simulink model "P2_SIL_Model_Diag"  (R2016a)
settings: Solver=ode2  StartTime=0.0  StopTime=Cycle_End  RelTol=1e-3
undefined symbols (not defined in the file): air, APP1_OOR, APP2_OOR, APP_Conversion_IN, APP_Mismatch, bms_inletair_temp, bms_maxchargecurrent, bms_maxdischargecurrent, BMS_Notfallkuehlung, BPP_Flt, cal, clt, ClutchEngag, CrankRequest, dcdc, eng, Engine, EngOverTemp, ENGTRQ_MSMCH_Degraded_CP, ENGTRQ_MSMCH_ErrCritical_CP, ENGTRQ_MSMCH_LimpHome_CP, EngTrqMismatch, env, ess, ESS, ESSOverTemp, fd, FFD, g, gb, Grade, IMG, KeyPos_Flt, KeyPosition, lib_APP_Conversion_IN, lib_ESS_plant_V1_2, lib_OBC_Manager, LossCAN, max_vehicle_rad_air_flow, MCUOverTemp, mot, MotDirMismatch, MotOverTemp, MotTrqMismatch, mph2kph, mph2ms, NeutralGear, obc, OBC_Manager, ParkGear, PRNDL_Flt, ReverseGear, RFD, rho, ShiftLeverPosition, sigbuilder_block, Speed, t_amb, time, tloop ... (+2)
libraries: simulink x104, EC2_libraries x12, Diagnostic x11, lib_CANerror_Detect x3, Utility x1
(part 4 of 11)

== system P2_SIL_Model_Diag/Camaro Plant Model/On-Board Charger/Soft_OBC/NLG5_ERR ==
  Bus Creator : BusCreator  Inputs=34
  Constant{1..34} (34 alike) : Constant  Value=0
  NLG5_ERR : Outport
  wires:
  Constant34/1 -> Bus Creator/34  "NLG5_E_PL_MV"
  Constant33/1 -> Bus Creator/33  "NLG5_E_PL_BV"
  Constant32/1 -> Bus Creator/32  "NLG5_E_PL_IT"
  Constant31/1 -> Bus Creator/31  "NLG5_E_C_VOR"
  Constant30/1 -> Bus Creator/30  "NLG5_E_C_TX"
  Constant29/1 -> Bus Creator/29  "NLG5_E_C_RX"
  Constant28/1 -> Bus Creator/28  "NLG5_E_SDT_BT"
  Constant27/1 -> Bus Creator/27  "NLG5_E_SDT_BV"
  Constant26/1 -> Bus Creator/26  "NLG5_E_SDT_AH"
  Constant25/1 -> Bus Creator/25  "NLG5_E_SDT_CT"
  Constant24/1 -> Bus Creator/24  "NLG5_E_F_CRC"
  Constant23/1 -> Bus Creator/23  "NLG5_E_NV_CRC"
  Constant22/1 -> Bus Creator/22  "NLG5_E_ES_CRC"
  Constant21/1 -> Bus Creator/21  "NLG5_E_EP_CRC"
  Constant20/1 -> Bus Creator/20  "NLG5_E_WDT"
  Constant19/1 -> Bus Creator/19  "NLG5_E_INIT"
  Constant18/1 -> Bus Creator/18  "NLG5_E_C_TO"
  Constant17/1 -> Bus Creator/17  "NLG5_E_C_OFF"
  Constant16/1 -> Bus Creator/16  "NLG5_E_B_P"
  Constant15/1 -> Bus Creator/15  "NLG5_E_T_C"
  Constant14/1 -> Bus Creator/14  "NLG5_E_T_POW"
  Constant13/1 -> Bus Creator/13  "NLG5_E_T_DIO"
  Constant12/1 -> Bus Creator/12  "NLG5_E_T_TR"
  Constant11/1 -> Bus Creator/11  "NLG5_E_T_EXT1"
  Constant10/1 -> Bus Creator/10  "NLG5_E_T_EXT2"
  Constant9/1 -> Bus Creator/9  "NLG5_E_T_EXT3"
  Constant8/1 -> Bus Creator/8  "NLG5_E_OOV"
  Constant7/1 -> Bus Creator/7  "NLG5_E_MOV_I"
  Constant5/1 -> Bus Creator/6  "NLG5_E_MOV_II"
  Constant2/1 -> Bus Creator/3  "NLG5_E_P_MV"
  Constant3/1 -> Bus Creator/4  "NLG5_E_P_OM"
  Constant1/1 -> Bus Creator/2  "NLG5_E_OF"
  Constant6/1 -> Bus Creator/1  "NLG5_E_MF"
  Bus Creator/1 -> NLG5_ERR/1  "NLG5_ERR"
  Constant4/1 -> Bus Creator/5  "NLG5_E_SC"

== system P2_SIL_Model_Diag/Camaro Plant Model/On-Board Charger/Soft_OBC/NLG5_ST ==
  Bus Creator : BusCreator  Inputs=24
  Constant10 : Constant
  Constant11 : Constant
  Constant{3..5,7,15..24} (14 alike) : Constant  Value=0
  Constant9 : Constant
  EVSE_Voltage : Constant  Value=obc.plant.init.Level2ChargerVoltage
  EVSE_Voltage1 : Constant  Value=obc.plant.init.Level1ChargerVoltage
  Logical Operator : Logic  Operator=OR  AllPortsSameDT=off  OutDataTypeStr=boolean
  Relational Operator : RelationalOperator  Operator===  OutDataTypeStr=boolean
  Relational Operator1 : RelationalOperator  Operator===  OutDataTypeStr=boolean
  NLG5_ST : Outport
  wires:
  EVSE_Voltage1/1 -> Relational Operator1/2
  EVSE_Voltage/1 -> Relational Operator/2
  [NLG5_MV_ACT] -> Relational Operator1/1, Relational Operator/1
  Constant4/1 -> Bus Creator/5  "NLG5_S_FAN"
  Bus Creator/1 -> NLG5_ST/1  "NLG5_ST"
  Logical Operator/1 -> Bus Creator/1  "NLG5_S_CP_DT"
  Relational Operator/1 -> Bus Creator/2, Logical Operator/1  "NLG5_S_UM_II"
  Constant3/1 -> Bus Creator/4  "NLG5_S_EUM"
  Relational Operator1/1 -> Bus Creator/3, Logical Operator/2  "NLG5_S_UM_I"
  Constant5/1 -> Bus Creator/6  "NLG5_S_WAR"
  Constant7/1 -> Bus Creator/7  "NLG5_S_ERR"
  [NLG5_S_HE] -> Bus Creator/8  "NLG5_S_HE"
  Constant9/1 -> Bus Creator/9  "NLG5_S_L_PMAX"
  Constant10/1 -> Bus Creator/10  "NLG5_S_L_CP"
  Constant11/1 -> Bus Creator/11  "NLG5_S_L_PI"
  [NLG5_S_L_MC] -> Bus Creator/12  "NLG5_S_L_MC"
  [NLG5_S_L_OC] -> Bus Creator/13  "NLG5_S_L_OC"
  [NLG5_S_L_OV] -> Bus Creator/14  "NLG5_S_L_OV"
  Constant15/1 -> Bus Creator/15  "NLG5_S_BPD_II"
  Constant16/1 -> Bus Creator/16  "NLG5_S_BPD_I"
  Constant17/1 -> Bus Creator/17  "NLG5_S_L_T_BATT"
  Constant18/1 -> Bus Creator/18  "NLG5_S_L_T_TR"
  Constant19/1 -> Bus Creator/19  "NLG5_S_L_T_DIO"
  Constant20/1 -> Bus Creator/20  "NLG5_S_L_T_POW"
  Constant21/1 -> Bus Creator/21  "NLG5_S_L_T_CPRIM"
  Constant22/1 -> Bus Creator/22  "NLG5_S_L_MO_MAX"
  Constant23/1 -> Bus Creator/23  "NLG5_S_L_OC_MAX"
  Constant24/1 -> Bus Creator/24  "NLG5_S_L_MC_MAX"

== system P2_SIL_Model_Diag/Camaro Plant Model/On-Board Charger/Soft_OBC/NLG5_TEMP ==
  Bus Creator : BusCreator  Inputs=4
  NoiseAdd : Subsystem  AncestorBlock=EC2_libraries/NoiseAdd  mask{variance=0, seed=0}
  NoiseAdd1 : Subsystem  AncestorBlock=EC2_libraries/NoiseAdd  mask{variance=0, seed=0}
  NoiseAdd2 : Subsystem  AncestorBlock=EC2_libraries/NoiseAdd  mask{variance=0, seed=0}
  NLG5_TEMP : Outport
  wires:
  Bus Creator/1 -> NLG5_TEMP/1  "NLG5_TEMP"
  [NLG5_TEMP] -> Bus Creator/1  "NLG5_P_TMP"
  [NLG5_TEMP] -> NoiseAdd/1(In)  "NLG5_TMP_EXT1"
  [NLG5_TEMP] -> NoiseAdd2/1(In)  "NLG5_TMP_EXT3"
  [NLG5_TEMP] -> NoiseAdd1/1(In)  "NLG5_TEMP_EXT2"
  NoiseAdd/1(Out) -> Bus Creator/2  "NLG5_TMP_EXT1"
  NoiseAdd1/1(Out) -> Bus Creator/3  "NLG5_TMP_EXT2"
  NoiseAdd2/1(Out) -> Bus Creator/4  "NLG5_TMP_EXT3"

== system P2_SIL_Model_Diag/Camaro Plant Model/On-Board Charger/Soft_OBC/VoltageEnable ==
  OV_COM : Inport
  Logical Operator1 : Logic  AllPortsSameDT=off  OutDataTypeStr=boolean
  MaxOutVoltage : Constant  Value=obc.plant.init.Maximum_Voltage_Out
  MinMax1 : MinMax  Inputs=2
  MinOutVoltage : Constant  Value=obc.plant.init.Minimum_Voltage_Out
  Relational Operator : RelationalOperator  OutDataTypeStr=boolean
  Relational Operator1 : RelationalOperator  Operator=<=  OutDataTypeStr=boolean
  Relational Operator2 : RelationalOperator  Operator=>  OutDataTypeStr=boolean
  VoltageEnable : Outport
  tag scope: NLG5_S_L_OV=global
  wires:
  MinMax1/1 -> Relational Operator/1
  MaxOutVoltage/1 -> MinMax1/2, Relational Operator2/2
  OV_COM/1 -> MinMax1/1, Relational Operator2/1
  Relational Operator1/1 -> Logical Operator1/2
  Relational Operator/1 -> Logical Operator1/1
  MinOutVoltage/1 -> Relational Operator1/1
  Relational Operator2/1 -> [NLG5_S_L_OV]
  Logical Operator1/1 -> VoltageEnable/1
  [NLG5_OV_ACT] -> Relational Operator/2, Relational Operator1/2

== system P2_SIL_Model_Diag/Camaro Plant Model/Transmission1/Inputs/Analog_fromHCU ==
  Outputs : Outport
  wires:
  [Analog] -> Outputs/1

== system P2_SIL_Model_Diag/Camaro Plant Model/Transmission1/Inputs/CAN_fromHCU ==
  Outputs : Outport
  wires:
  [HCU_to_VEH_CAN] -> Outputs/1

== system P2_SIL_Model_Diag/Camaro Plant Model/Transmission1/Inputs/Digital_fromHCU ==
  Outputs : Outport
  wires:
  [Digital] -> Outputs/1

== system P2_SIL_Model_Diag/Camaro Plant Model/Transmission1/Soft TCM/6L45 Logic/Gearbox_Control.Shift_Schedule.PlotShiftSchedule ==
  f : TriggerPort  TriggerType=function-call  VariantControl=Variant
      settings: CopyFcn=Stateflow.SLINSF.SimulinkMan.removeBlockPreDeleteFcn  PreDeleteFcn=Stateflow.SLINSF.SimulinkMan.unsafePredeleteFcn
  Subsystem : Subsystem
      settings: OpenFcn=|
      | figure;
      | PlotGearShiftSchedule(Gearbox.L45.PedalPositions,Gearbox.L45.UpShiftSpeeds,Gearbox.L45.DownShiftSpeeds,'6L45')
      mask Display: disp('Plot')

== system P2_SIL_Model_Diag/Camaro Plant Model/Transmission1/Soft TCM/6L45 Logic/Gearbox_Control.Shift_Schedule.calc_down ==
  Gear : Inport
  APP : Inport  Port=2
  f : TriggerPort  TriggerType=function-call  VariantControl=Variant
      settings: CopyFcn=Stateflow.SLINSF.SimulinkMan.removeBlockPreDeleteFcn  PreDeleteFcn=Stateflow.SLINSF.SimulinkMan.unsafePredeleteFcn
  Calculate Downshift Threshold : Lookup2D  RowIndex=gb.ctrl.dmd.init.gear_dnshift.idx1_lin_accel  ColumnIndex=[2,3,4,5,6,7,8]  Table=gb.ctrl.dmd.init.gear_dnshift.map'  LookUpMeth=Interpolation-Use End Values
  down_th : Outport
  wires:
  APP/1 -> Calculate Downshift Threshold/1
  Gear/1 -> Calculate Downshift Threshold/2
  Calculate Downshift Threshold/1 -> down_th/1

== system P2_SIL_Model_Diag/Camaro Plant Model/Transmission1/Soft TCM/6L45 Logic/Gearbox_Control.Shift_Schedule.calc_up ==
  Gear : Inport
  APP : Inport  Port=2
  f : TriggerPort  TriggerType=function-call  VariantControl=Variant
      settings: CopyFcn=Stateflow.SLINSF.SimulinkMan.removeBlockPreDeleteFcn  PreDeleteFcn=Stateflow.SLINSF.SimulinkMan.unsafePredeleteFcn
  Calculate Upshift Threshold : Lookup2D  RowIndex=gb.ctrl.dmd.init.gear_upshift.idx1_lin_accel  ColumnIndex=[1,2,3,4,5,6,7]  Table=gb.ctrl.dmd.init.gear_upshift.map'  LookUpMeth=Interpolation-Use End Values
  up_th : Outport
  wires:
  Gear/1 -> Calculate Upshift Threshold/2
  APP/1 -> Calculate Upshift Threshold/1
  Calculate Upshift Threshold/1 -> up_th/1

== system P2_SIL_Model_Diag/Camaro Plant Model/Transmission1/Soft TCM/6L45 Logic/Torque_Converter_Control.calc_lockup ==
  Gear : Inport
  APP : Inport  Port=2
  f : TriggerPort  TriggerType=function-call  VariantControl=Variant
      settings: CopyFcn=Stateflow.SLINSF.SimulinkMan.removeBlockPreDeleteFcn  PreDeleteFcn=Stateflow.SLINSF.SimulinkMan.unsafePredeleteFcn
  Calculate Lockup Threshold : Lookup2D  RowIndex=cpl.ctrl.init.trqconv_lockup.idx1_lin_accel  ColumnIndex=cpl.ctrl.init.trqconv_lockup.idx2_gear  Table=cpl.ctrl.init.trqconv_lockup.map  LookUpMeth=Interpolation-Use End Values
  lockup_th : Outport
  wires:
  Gear/1 -> Calculate Lockup Threshold/2
  APP/1 -> Calculate Lockup Threshold/1
  Calculate Lockup Threshold/1 -> lockup_th/1

== system P2_SIL_Model_Diag/Camaro Plant Model/Transmission1/Soft TCM/6L45 Logic/Torque_Converter_Control.calc_unlock ==
  Gear : Inport
  APP : Inport  Port=2
  f : TriggerPort  TriggerType=function-call  VariantControl=Variant
      settings: CopyFcn=Stateflow.SLINSF.SimulinkMan.removeBlockPreDeleteFcn  PreDeleteFcn=Stateflow.SLINSF.SimulinkMan.unsafePredeleteFcn
  Calculate Unlock Threshold : Lookup2D  RowIndex=cpl.ctrl.init.trqconv_unlock.idx1_lin_accel  ColumnIndex=cpl.ctrl.init.trqconv_unlock.idx2_gear  Table=cpl.ctrl.init.trqconv_unlock.map  LookUpMeth=Interpolation-Use End Values
  unlock_th : Outport
  wires:
  Gear/1 -> Calculate Unlock Threshold/2
  APP/1 -> Calculate Unlock Threshold/1
  Calculate Unlock Threshold/1 -> unlock_th/1

== system P2_SIL_Model_Diag/Camaro Plant Model/Transmission1/Transmission Plant/ Actuators ==
  In1 : Inport
  Bus Selector : BusSelector  OutputSignals=TransEstGear,LockupCmd
  Out2 : Outport
  Out5 : Outport  Port=2
  wires:
  Bus Selector/2 -> Out5/1  "<LockupCmd>"
  Bus Selector/1 -> Out2/1  "<TransEstGear>"
  In1/1 -> Bus Selector/1

== system P2_SIL_Model_Diag/Camaro Plant Model/Transmission1/Transmission Plant/Gearbox ==
  TransEstGear : Inport
  gb_trq_in gb_inertia_in : Inport  Port=2
  gb_spd_out : Inport  Port=3
  Bus Creator : BusCreator  Inputs=2
  Bus Selector : BusSelector  OutputSignals=tc_trq_out,tc_inertia_out
  Gear : Lookup  InputValues=gb.plant.init.gear.idx1_shifter  Table=gb.plant.init.gear.idx2_gear  LookUpMeth=Interpolation-Use End Values  OutDataTypeStr=double  SaturateOnIntegerOverflow=on
  Inertia Calculation : Subsystem
  Memory : Memory
  Speed Calculation : Subsystem
  Torque calculation : Subsystem
  gear ratio table : Lookup  InputValues=gb.plant.init.ratio.idx1_gear  Table=gb.plant.init.ratio.map  LookUpMeth=Interpolation-Use End Values  SaturateOnIntegerOverflow=on
  gb_trq_out gb_inertia_out : Outport
  gb_spd_in : Outport  Port=2
  tag scope: gb_gear=global, gb_inertia_in=global, gb_inertia_out=global, gb_spd_in=global, gb_spd_out=global, gb_trq_in=global, gb_trq_out=global, gb_trq_ratio=global
  wires:
  TransEstGear/1 -> Memory/1
  Bus Selector/1 -> [gb_trq_in], Speed Calculation/3(torque input), Torque calculation/3(" input torque")  "<tc_trq_out>"
  Gear/1 -> Speed Calculation/1(gear number), [gb_gear], gear ratio table/1, Inertia Calculation/2(gear number), Torque calculation/2(gear number)
  Torque calculation/1(torque_out) -> Bus Creator/1, [gb_trq_out]  "gb_trq_out"
  gb_spd_out/1 -> Torque calculation/1(speed out), [gb_spd_out], Speed Calculation/2(spd out)
  gb_trq_in gb_inertia_in/1 -> Bus Selector/1
  Speed Calculation/1(Speed) -> [gb_spd_in], gb_spd_in/1
  Bus Selector/2 -> [gb_inertia_in], Inertia Calculation/1(Inertia_in), Speed Calculation/4(Inertia Input)  "<tc_inertia_out>"
  Inertia Calculation/1(Inertia) -> [gb_inertia_out], Bus Creator/2  "gb_inertia_out"
  Bus Creator/1 -> gb_trq_out gb_inertia_out/1
  gear ratio table/1 -> [gb_trq_ratio]
  Memory/1 -> Gear/1

== system P2_SIL_Model_Diag/Camaro Plant Model/Transmission1/Transmission Plant/Sensors ==
  In2 : Inport
  In3 : Inport  Port=2
  In4 : Inport  Port=3
  In5 : Inport  Port=4
  In6 : Inport  Port=5
  In7 : Inport  Port=6
  Bus Creator : BusCreator  Inputs=6
  Out1 : Outport
  wires:
  In7/1 -> Bus Creator/6  "TrnsOutShftTrq"
  In6/1 -> Bus Creator/5  "TrnsOutShftAngVel"
  In3/1 -> Bus Creator/2  "turbine_spd_rads"
  In5/1 -> Bus Creator/4  "tc_trq_out"
  In4/1 -> Bus Creator/3  "tc_trq_in"
  In2/1 -> Bus Creator/1  "impeller_spd_rads"
  Bus Creator/1 -> Out1/1

== system P2_SIL_Model_Diag/Camaro Plant Model/Transmission1/Transmission Plant/Torque Converter ==
  tc_lockup : Inport
  tc_shaft_in : Inport  Port=2
  tc_spd_out : Inport  Port=3
  Bus Creator : BusCreator  Inputs=2
  Bus Selector : BusSelector  OutputSignals=mot_trq_out,mot_inertia_out
  Inertia Calculation : Subsystem
  Speed Calculation : Subsystem
  Torque Calculation : Subsystem
  tc_shaft_out : Outport
  cpl_spd_in : Outport  Port=2
  tag scope: tc_spd_in=global, tc_spd_out=global, tc_trq_in=global, tc_trq_out=global
  wires:
  Torque Calculation/2(turbine_trq) -> Bus Creator/1, [tc_trq_out]  "tc_trq_out"
  Torque Calculation/1("impeller_trq ") -> Speed Calculation/4(impeller_trq)
  Speed Calculation/1(impeller spd) -> [tc_spd_in], Torque Calculation/1("impeller_spd "), cpl_spd_in/1
  Inertia Calculation/2(impeller inertia) -> Speed Calculation/2(impeller_inertia)
  Inertia Calculation/1(turbine inertia) -> Bus Creator/2  "tc_inertia_out"
  tc_spd_out/1 -> Torque Calculation/2(turbine_spd), Speed Calculation/1(turbine_spd), [tc_spd_out]
  tc_shaft_in/1 -> Bus Selector/1
  Bus Creator/1 -> tc_shaft_out/1
  Bus Selector/1 -> [tc_trq_in], Torque Calculation/4(input_trq)  "<mot_trq_out>"
  Bus Selector/2 -> Inertia Calculation/1(inertia in)  "<mot_inertia_out>"
  tc_lockup/1 -> Speed Calculation/3(lockup_cmd), Inertia Calculation/2(lockup cmd), Torque Calculation/3(lockup_cmd)  "tc_lockup_cmd"

== system P2_SIL_Model_Diag/Camaro Plant Model/Wheels/Force calculation/Blending ==
  note: State dependent blending
  input : Inport
  Control (state) : Inport  Port=2
  Fcn : Fcn  Expr=(u<xl)*yl + (xl<=u)*(u<xc)*((yc-yl)*(u-xl)/(xc-xl)+yl) + (xc<=u)*(u<xr)*((yc-yr)*(u-xr)/(xc-xr)+yr) + (xr<=u)*yr
  Product : Product  SaturateOnIntegerOverflow=on  InputSameDT=on  OutDataTypeStr=Inherit: Same as first input
  Out1 : Outport
  wires:
  input/1 -> Product/1
  Control (state)/1 -> Fcn/1
  Product/1 -> Out1/1
  Fcn/1 -> Product/2

== system P2_SIL_Model_Diag/Camaro Plant Model/Wheels/Force calculation/Rolling Resistance ==
  whl_spd : Inport
  grade : Inport  Port=2
  Add : Sum  Inputs=++++
  Add1 : Sum
  Divide : Product  Inputs=*/
  Product : Product  Inputs=3  SaturateOnIntegerOverflow=on  InputSameDT=on  OutDataTypeStr=Inherit: Same as first input
  Product{1..4,7} (5 alike) : Product  RndMeth=Zero
  Product5 : Product  Inputs=3  RndMeth=Zero
  Product6 : Product  Inputs=5  RndMeth=Zero
  Relational Operator : RelationalOperator  Operator=<=  InputSameDT=on
  Relational Operator1 : RelationalOperator  Operator=>  InputSameDT=on
  Sign : Signum
  Trigonometric Function : Trigonometry  Operator=cos
  env.init.gravity : Constant  Value=g
  radius : Gain  Gain=whl.plant.init.radius  SaturateOnIntegerOverflow=on  OutDataTypeStr=Inherit: Same as input  ParamDataTypeStr=Inherit: Same as input
  veh.plant.init.mass.total : Constant  Value=chas.plant.init.mass.body
  whl.plant.calc.weight_fraction_effective : Constant
  whl.plant.init.coeff_roll1 : Constant  Value=whl.plant.init.coeff_roll1
  whl.plant.init.coeff_roll2 : Constant  Value=whl.plant.init.coeff_roll2
  whl.plant.init.coeff_roll3 : Constant  Value=whl.plant.init.coeff_roll3
  whl.plant.init.coeff_roll4 : Constant  Value=whl.plant.init.coeff_roll4
  whl.plant.init.spd_thresh : Constant  Value=whl.plant.init.spd_thresh
  rolling resistence : Outport
  wires:
  Product/1 -> radius/1
  Sign/1 -> Product/3
  radius/1 -> rolling resistence/1  "tire rollig resistance"
  whl.plant.init.coeff_roll2/1 -> Product1/2
  whl.plant.init.coeff_roll3/1 -> Product2/2
  whl.plant.init.coeff_roll4/1 -> Product3/2
  whl_spd/1 -> Sign/1, Relational Operator/1, Product7/1, Relational Operator1/1, Product1/1, Product4/1, Product4/2, Product5/1, Product5/2, Product5/3
  Product4/1 -> Product2/1
  Product5/1 -> Product3/1
  Product3/1 -> Add/1
  Product2/1 -> Add/2
  Product1/1 -> Add/3
  whl.plant.init.coeff_roll1/1 -> Add/4
  Add/1 -> Product6/2
  veh.plant.init.mass.total/1 -> Product6/3
  env.init.gravity/1 -> Product6/4
  whl.plant.calc.weight_fraction_effective/1 -> Product6/5
  Trigonometric Function/1 -> Product6/1
  grade/1 -> Trigonometric Function/1
  Product6/1 -> Product/1
  whl.plant.init.spd_thresh/1 -> Relational Operator/2, Divide/2, Relational Operator1/2
  Relational Operator/1 -> Product7/2
  Product7/1 -> Divide/1
  Divide/1 -> Add1/1
  Relational Operator1/1 -> Add1/2
  Add1/1 -> Product/2

== system P2_SIL_Model_Diag/Controller/HSC/Camaro Fault Detection/Component Diagnostic ==
  note: Component Status Setting Rule
      | xxx_CompStatus could be 0, 1, 2 or 3
      | 0: component needs to be offline
      | 1: component needs torque plant to deliver creep torque
      | 2: component needs torque plant to limit maximum torque delivery
      | 3: component needs torque plant to operate normally
  note: Component Diagnostics
  Sensors1 : Inport
  Bus Creator : BusCreator  Inputs=9
  Clutch Component Diagnostic : Subsystem
  Driver Input Diagnostic : Subsystem
  ESS Component Diagnostic : Subsystem
  Engine Component Diagnostic : Subsystem
  Motor Component Diagnostic : Subsystem
  Override Clutch Status : Subsystem  AncestorBlock=Diagnostic/Camaro Diagnostic/Input Conversions/DriverInput_Conversions/Override APP (%)
  Override Driver Status : Subsystem  AncestorBlock=Diagnostic/Camaro Diagnostic/Input Conversions/DriverInput_Conversions/Override APP (%)
  Override ESS Status : Subsystem  AncestorBlock=Diagnostic/Camaro Diagnostic/Input Conversions/DriverInput_Conversions/Override APP (%)
  Override Engine Status : Subsystem  AncestorBlock=Diagnostic/Camaro Diagnostic/Input Conversions/DriverInput_Conversions/Override APP (%)
  Override MCU Status : Subsystem  AncestorBlock=Diagnostic/Camaro Diagnostic/Input Conversions/DriverInput_Conversions/Override APP (%)
  Override TCM Status : Subsystem  AncestorBlock=Diagnostic/Camaro Diagnostic/Input Conversions/DriverInput_Conversions/Override APP (%)
  Transmission Component Diagnostic : Subsystem
  Out2 : Outport
  wires:
  Sensors1/1 -> Driver Input Diagnostic/1(In1), ESS Component Diagnostic/1(In1), Bus Creator/9, Clutch Component Diagnostic/1(In1), Transmission Component Diagnostic/1(In1), Engine Component Diagnostic/1(In1), Motor Component Diagnostic/1(In1)  "RawSig"
  Bus Creator/1 -> Out2/1
  Driver Input Diagnostic/1(Out1) -> Override Driver Status/1(In1)  "Diver_CompDiag"
  ESS Component Diagnostic/1(Out1) -> Override ESS Status/1(In1)  "ESS_CompDiag"
  Engine Component Diagnostic/1(Out1) -> Override Engine Status/1(In1)  "ECM_CompDiag"
  Transmission Component Diagnostic/1(Out1) -> Override TCM Status/1(In1)  "TCM_CompDiag"
  Clutch Component Diagnostic/1(Out1) -> Override Clutch Status/1(In1)  "Clutch_Component"
  Override ESS Status/1(Out1) -> Bus Creator/2  "BMS_Status"
  Override Engine Status/1(Out1) -> Bus Creator/5  "ECM_Status"
  Override TCM Status/1(Out1) -> Bus Creator/7  "TCM_Status"
  Override Clutch Status/1(Out1) -> Bus Creator/8  "Clutch_Status"
  Override Driver Status/1(Out1) -> Bus Creator/1  "Driver_Input_Status"
  Engine Component Diagnostic/2(Out2) -> Bus Creator/6
  Motor Component Diagnostic/1(Out1) -> Override MCU Status/1(In1)  "MCU_CompDiag"
  Override MCU Status/1(Out1) -> Bus Creator/3  "MCU_Status"
  Motor Component Diagnostic/2(Out2) -> Bus Creator/4

== system P2_SIL_Model_Diag/Controller/HSC/Camaro Fault Detection/Input Conversions ==
  note: Input Conversions and Override Switches
  note: These subsystems convert variable types to match those used in the
      | supervisor. In addition, override switches installed on each signal can
      | be used to manually override and signal for testing purposes
  RawSig : Inport
  BMS_Conversions : Subsystem
  Bus Creator : BusCreator  Inputs=7
  Clutch_Conversions : Subsystem
  DriverInput_Conversions : Subsystem
  ECM_Conversions : Subsystem
  MCU_Conversions : Subsystem
  TCM_Conversions : Subsystem
  VehSig : Outport
  wires:
  DriverInput_Conversions/1(Out1) -> Bus Creator/1
  Bus Creator/1 -> VehSig/1  "InputConvAndOvrd"
  MCU_Conversions/1(Out1) -> Bus Creator/3
  BMS_Conversions/1(Out1) -> Bus Creator/2
  RawSig/1 -> DriverInput_Conversions/1(In1), BMS_Conversions/1(In1), Clutch_Conversions/1(In1), Bus Creator/7, TCM_Conversions/1(In1), ECM_Conversions/1(In1), MCU_Conversions/1(In1)  "RawSig"
  ECM_Conversions/1(Out1) -> Bus Creator/4
  TCM_Conversions/1(Out1) -> Bus Creator/5
  Clutch_Conversions/1(Out1) -> Bus Creator/6

== system P2_SIL_Model_Diag/Controller/HSC/Camaro Fault Detection/Signal Diagnostic ==
  note: Signal Valid Setting Rule
      | xxx_yyy_[z]_SigValid could be 0 or 1
      | 0: signal invalid
      | 1: signal vaild
  note: Signal Naming Rule
      | Example: xxx_yyy_[z]_SigValid
      | xxx: source of the signal (Drv, Clu, BCM, ECM, TCM, BMS and MCU)
      | yyy: description of the signal
      | z: unit of the signal (V, A, Nm, m/s, %, 01, 0123, etc.)
  note: These subsystems evaluate each signal for proper value range and other checks
  note: Signal Diagnostics
  VehSig : Inport
  Bus Creator : BusCreator  Inputs=6
  Clutch Signal Diagnostic : Subsystem  AncestorBlock=Diagnostic/Camaro Diagnostic/Signal Diagnostic/Transmission Signal Diagnostic
  Driver Signal Diagnostic : Subsystem
  ESS Signal Diagnostic : Subsystem
  Engine Signal Diagnostic : Subsystem
  Motor Signal Diagnostic : Subsystem
  Transmission Signal Diagnostic : Subsystem
  Out2 : Outport
  wires:
  VehSig/1 -> Driver Signal Diagnostic/1(Sensors1), ESS Signal Diagnostic/1(Sensors1), Motor Signal Diagnostic/1(Sensors1), Clutch Signal Diagnostic/1(Sensors1), Transmission Signal Diagnostic/1(Sensors1), Engine Signal Diagnostic/1(Sensors1)
  Driver Signal Diagnostic/1(Driver_SigDiag) -> Bus Creator/1  "Driver_SigDiag"
  ESS Signal Diagnostic/1(ESS_SigDiag) -> Bus Creator/2  "ESS_SigDiag"
  Motor Signal Diagnostic/1(Motor_SigDiag) -> Bus Creator/3  "Motor_SigDiag"
  Engine Signal Diagnostic/1(Engine_SigDiag) -> Bus Creator/4  "Engine_SigDiag"
  Transmission Signal Diagnostic/1(Out2) -> Bus Creator/5  "Transmission_SigDiag"
  Bus Creator/1 -> Out2/1  "SignalDiag"
  Clutch Signal Diagnostic/1(Out2) -> Bus Creator/6  "Clutch_SigDiag"

== system P2_SIL_Model_Diag/Controller/HSC/Camaro Fault Detection/Signal Generator  ==
  note: Signal Generator
  BCM_APM_OBC_CANFault : lib_CANerror_Detect/CAN_Error_Detection/BCM_APM_OBC_CANFault  Commented=on
  BMS_Signals : Subsystem
  Bus Creator2 : BusCreator  Inputs=6
  Clutch_Signals : Subsystem
  Driver_Signals : Subsystem
  EBCM_BodyCM_CANFault : lib_CANerror_Detect/CAN_Error_Detection/EBCM_BodyCM_CANFault  Commented=on
  ECM_Signals : Subsystem
  ECM_TCM_CANFault : lib_CANerror_Detect/CAN_Error_Detection/ECM_TCM_CANFault  Commented=on
  MCU_Signals : Subsystem
  TCM_Signals : Subsystem
  Out1 : Outport
  wires:
  [BMS_Signals] -> Bus Creator2/1
  [Driver_Signals] -> Bus Creator2/2
  Bus Creator2/1 -> Out1/1
  [MCU_Signals] -> Bus Creator2/3
  [ECM_Signals] -> Bus Creator2/4
  [TCM_Signals] -> Bus Creator2/5
  [Clutch_Signals] -> Bus Creator2/6
  EBCM_BodyCM_CANFault/1 -> ?
  ECM_TCM_CANFault/1 -> ?
  BCM_APM_OBC_CANFault/1 -> ?

== system P2_SIL_Model_Diag/Controller/HSC/Camaro Fault Detection/SystemDiag ==
  note: 0: SystemStatus: Offline
      | 1: SystemStatus Online
      | 2: SystemStatus Limited
  note: Powertrain Diagnostics
  note: These subsystems evaluate each powertrain to determine
      | the level of functionality allowed based on each of its components.
  In1 : Inport
  Bus Creator : BusCreator  Inputs=4
  Combined_SystemDiagnostics : Subsystem  Commented=through
  eSystemDiagnostics : Subsystem
  iceSystemDiagnostics : Subsystem
  Out1 : Outport
  wires:
  eSystemDiagnostics/1(Out1) -> Bus Creator/1
  Bus Creator/1 -> Out1/1  "SystemDiag"
  In1/1 -> eSystemDiagnostics/1(In1), iceSystemDiagnostics/1(In1), Bus Creator/4  "CompSig"
  iceSystemDiagnostics/1(Out1) -> Bus Creator/2

== system P2_SIL_Model_Diag/Controller/HSC/Driver_Requests/APP_BPP to DrvIntndAxlTrq1 ==
  note: //*cal.RWD.CreepTrqEnableBPP*//
  note: $Author: fj4499 $
      | $Rev: 577 $
      | $Date: 2016-09-19 08:53:15 -0500 (Mon,19 Sep 2016) $
  Sensors : Inport
  Abs : Abs
  Bus Creator : BusCreator  Inputs=3
  Bus Selector : BusSelector  OutputSignals=from_Analog.drv_APP_req_[%],from_CAN.fromVEH_CAN.from_TCM.Ratio,from_CAN.fromVEH_CAN.from_BCM.BrkPdlPos,from_CAN.fromEBCAN.from_ECM.VehSpdAvgDrvn,from_CAN.fromHV_CAN.from_MCU.D2_Motor_Speed
  Compare To Constant1 : simulink/Logic and Bit Operations/Compare To Constant  relop=>=  const=10  OutDataTypeStr=boolean
  Constant : Constant  Value=0
  Constant2 : Constant  Value=0
  MotorCreepTrq : Lookup  InputValues=cal.RWD.CreepTrq.idx1_spd  Table=cal.RWD.CreepTrq.idx2_trq
  Post Driver Intnded Axle Torque : Subsystem
  Scope : Scope
  Sum : Sum
  Sum1 : Sum
  Switch1 : Switch  Threshold=cal.Regen.MinMotSpd
  Switch2 : Switch  Criteria=u2 > Threshold  Threshold=1
  Switch3 : Switch  Threshold=1
  IntndAxlTrq : Outport
  IntndAxlTrqStatus : Outport  Port=2
  wires:
  Constant/1 -> Sum/1, Bus Creator/2  "BrkIntndAxlTrq"
  Abs/1 -> Switch1/2
  Bus Creator/1 -> IntndAxlTrqStatus/1
  Switch1/1 -> IntndAxlTrq/1
  Bus Selector/3 -> Compare To Constant1/1  "<BrkPdlPos>"
  Sum/1 -> Switch1/1, Bus Creator/1  "FullDrvIntndAxlTrq"
  Sensors/1 -> Bus Selector/1
  Post Driver Intnded Axle Torque/1(DrvIntndAxlTrq) -> Switch2/1, Sum1/1  "PostDrvIntndAxlTrq"
  Bus Selector/1 -> Post Driver Intnded Axle Torque/1(APP)  "<drv_APP_req_[%]>"
  Bus Selector/5 -> Abs/1  "<D2_Motor_Speed>"
  MotorCreepTrq/1 -> Switch3/3
  Sum1/1 -> Switch2/3
  Switch2/1 -> Scope/1, Switch1/3, Bus Creator/3, Sum/2  "DrvIntndAxlTrq"
  Bus Selector/4 -> MotorCreepTrq/1  "<VehSpdAvgDrvn>"
  Switch3/1 -> Sum1/2  "MotAxlCrpTrq"
  Compare To Constant1/1 -> Switch3/2
  Constant2/1 -> Switch3/1
  Bus Selector/2 -> Post Driver Intnded Axle Torque/2(TransGearRatio)  "<Ratio>"
  [mode] -> Post Driver Intnded Axle Torque/3(Mode), Switch2/2

== system P2_SIL_Model_Diag/Controller/HSC/Driver_Requests/APP_BPP to DrvIntndAxlTrq2 ==
  note: $Author: fj4499 $
      | $Rev: 577 $
      | $Date: 2016-09-19 08:53:15 -0500 (Mon,19 Sep 2016) $
  Sensors : Inport
  Bus Selector : BusSelector  OutputSignals=from_Analog.drv_APP_req_[%]
  Bus Selector1 : BusSelector  OutputSignals=DrvIntndAxlTrq
  Post Driver Intnded Axle Torque : Subsystem
  IntndAxlTrq : Outport
  wires:
  Bus Selector/1 -> Post Driver Intnded Axle Torque/1(APP)  "<drv_APP_req_[%]>"
  Sensors/1 -> Bus Selector/1
  [mode] -> Post Driver Intnded Axle Torque/3(Mode)
  Post Driver Intnded Axle Torque/1(DrvIntndAxlTrq) -> Bus Selector1/1
  Bus Selector1/1 -> IntndAxlTrq/1  "<DrvIntndAxlTrq>"
  [gb_trq_ratio] -> Post Driver Intnded Axle Torque/2(TransGearRatio)

== system P2_SIL_Model_Diag/Controller/HSC/Driver_Requests/Vehicle_Shutdown ==
  note: $Author: eo1000 $
      | $Rev: 509 $
      | $Date: 2014-01-13 11:43:00 -0500 (Mon, 13 Jan 2014) $
  note: Make sure PD is sent before components are disabled
  note: Key Position
      | KeyOFF: 0
      | KeyAccessory: 1
      | KeyIgnition: 2
      | KeyCrank = 3
  note: HCU Init: HCUStatus = 0;
      | Waiting Key OFF Cmd: HCUStatus = 1;
      | USB Diag Performed: HCUStatus = 2;
      | ECUs are off: HCUStatus = 3
      | CAN Off Cmd: HCUStatus = 4;
      | HCU Off Cmd: HCUStatus = 5;
  Sensors : Inport
  Diagnostics : Inport  Port=2
  Bus Selector : BusSelector  OutputSignals=from_CAN.fromVEH_CAN.from_BCM.SysPwrMd,from_Analog.EVSEPlugged
  Components Disabled : Subsystem
  Constant : Constant  Value=cal.Time.DiagUSB
  Gain2 : Gain  Gain=1/tloop
  HCU_Shutdown : Stateflow chart  TreatAsAtomicUnit=on
  HCUONCmd : Outport
  HCUStatus : Outport  Port=2
  Components_Disabled : Outport  Port=3
  wires:
  Bus Selector/2 -> HCU_Shutdown/4(Plugged)  "<EVSEPlugged>"
  HCU_Shutdown/1(HCUStatus) -> HCUStatus/1
  Sensors/1 -> Bus Selector/1, Components Disabled/1(Sensors)
  Components Disabled/1(Comp_Disabled) -> Components_Disabled/1, HCU_Shutdown/1(DisableComponents)
  Constant/1 -> Gain2/1
  Bus Selector/1 -> HCU_Shutdown/3(Key_Position)  "<SysPwrMd>"
  HCU_Shutdown/2(HCU_ON) -> HCUONCmd/1  "HCUONCmd"
  Gain2/1 -> HCU_Shutdown/2(DiagUSBTimerMax)
  Diagnostics/1 -> Components Disabled/2(Diagnostics)

== system P2_SIL_Model_Diag/Controller/HSC/Driver_Requests/Vehicle_Startup ==
  note: $Author: eo1000 $
      | $Rev: 294 $
      | $Date: 2013-11-14 10:23:49 -0500 (Thu, 14 Nov 2013) $
  note: DriverDoor <DOAjrSwAtv>
      | Open: 1
      | Close: 0
  note: SysPwrMd (EC3)
      | 0 - Off
      | 1 -  Accessory
      | 2 - Run
      | 3 - Crank Request
  Sensors : Inport
  Bus Creator : BusCreator  Inputs=2
  Enable Propulsion : Subsystem  RequirementInfo={'other' 'HCU_Requirements.xlsx' '@Simulink_requirement_item_9' 'true' 'Check if the conditions are true to allow regular or emergency (when in highway traffic) propulsion system activation ' '' } %GIDa_dfd30209_921a_4d0b_a7c1_96ecad5085d2
  Vehicle_Startup_Signals : Outport
  wires:
  Bus Creator/1 -> Vehicle_Startup_Signals/1
  Sensors/1 -> Enable Propulsion/1(Sensors)
  Enable Propulsion/1(StartVehEnable) -> Bus Creator/1  "EnablePrplsn"
  Enable Propulsion/2(EnablePrplsnStatus) -> Bus Creator/2  "EnablePrplsnStatus"

== system P2_SIL_Model_Diag/Controller/HSC/Powertrain Manager/HV Manager ==
  note: //OBC status to be coming from Diagnostic later//
  note: //add OBC charge limits//
  Sensors : Inport
  Controls : Inport  Port=2
  APM_Manager : Subsystem  Commented=on
  BMS_Manager : Subsystem
  OBC_Manager : Subsystem  AncestorBlock=lib_OBC_Manager/OBC_Manager
  BMS_CAN : Outport
  HV_BUS_Status : Outport  Port=2
  OBC_CAN : Outport  Port=3
  OBC_Status : Outport  Port=4
  BMS_Digital : Outport  Port=5
  APM_CAN : Outport  Port=6
  APM_Status : Outport  Port=7
  wires:
  BMS_Manager/2(HV_BUS_Status) -> [HV_BUS_Status], HV_BUS_Status/1  "HV_BUS_Status"
  Sensors/1 -> BMS_Manager/1(Sensors), OBC_Manager/2(Sensors)
  [HV_BUS_Status] -> OBC_Manager/1(HV_Status)
  OBC_Manager/1(OBC CAN) -> OBC_CAN/1
  OBC_Manager/2(OBC Status) -> OBC_Status/1
  Controls/1 -> BMS_Manager/2(Controls)
  BMS_Manager/1(BMS CAN) -> BMS_CAN/1
  BMS_Manager/3(BMS Digital) -> BMS_Digital/1
  [HV_BUS_Status] -> APM_Manager/1(HV_Status)
  APM_Manager/1(APM Controls) -> APM_CAN/1
  APM_Manager/2(APM Status) -> APM_Status/1

== system P2_SIL_Model_Diag/Controller/HSC/Powertrain Manager/Output Conversion ==
  In1 : Inport
  In2 : Inport  Port=2
  In3 : Inport  Port=3
  In4 : Inport  Port=4
  In5 : Inport  Port=5
  In6 : Inport  Port=6
  Bus Creator : BusCreator  Inputs=14
  Bus Creator1 : BusCreator  Inputs=7
  Bus Selector2 : BusSelector  OutputSignals=powerMode,closeMaincReq,EnablePrplsn,ClutchEngage,EngAppReq,EngOnReq,MtrTrqCmd,EnableInverter,EngTrqCmd,HV_req,SysPwrMd_0_3,TrnsShftLvrPos,VehSpdAvgDrvn_kph,AccPos_Perc
  Data Type Conversion{,1..3,5..13} (13 alike) : DataTypeConversion
  Memory : Memory
  Memory1 : Memory
  Memory2 : Memory
  Out1 : Outport
  wires:
  In1/1 -> [BMS_CAN]
  In2/1 -> [OBC_CAN]
  In4/1 -> Bus Selector2/1
  Bus Selector2/1 -> Memory/1  "<powerMode>"
  Bus Selector2/2 -> Memory1/1  "<closeMaincReq>"
  Bus Selector2/3 -> Data Type Conversion2/1  "<EnablePrplsn>"
  Bus Selector2/4 -> Data Type Conversion3/1  "<ClutchEngage>"
  Bus Selector2/6 -> Data Type Conversion5/1  "<EngOnReq>"
  Bus Selector2/7 -> Data Type Conversion6/1  "<MtrTrqCmd>"
  Bus Selector2/8 -> Data Type Conversion7/1  "<EnableInverter>"
  Bus Selector2/9 -> Data Type Conversion8/1  "<EngTrqCmd>"
  Bus Selector2/10 -> Data Type Conversion9/1  "<HV_req>"
  Bus Selector2/11 -> Memory2/1  "<SysPwrMd_0_3>"
  Data Type Conversion1/1 -> Bus Creator/2  "MO_BMS_Sollmodus"
  Data Type Conversion2/1 -> Bus Creator/3  "EnablePrplsn"
  Data Type Conversion3/1 -> Bus Creator/4  "ClutchEngage"
  Bus Selector2/5 -> Bus Creator/5  "<EngAppReq>"
  Data Type Conversion6/1 -> Bus Creator/7  "Torque_Command"
  Data Type Conversion7/1 -> Bus Creator/8  "Inverter_Enable"
  Data Type Conversion8/1 -> Bus Creator/9  "EngTrqCmd"
  Data Type Conversion9/1 -> Bus Creator/10  "HV_req"
  Data Type Conversion10/1 -> Bus Creator/11  "SysPwrMd"
  Data Type Conversion/1 -> Bus Creator/1  "powerMode"
  In3/1 -> [MCU_CAN]
  Data Type Conversion5/1 -> Bus Creator/6  "EngOnReq"
  Bus Creator1/1 -> Out1/1
  [BMS_CAN] -> Bus Creator1/1
  [OBC_CAN] -> Bus Creator1/2
  [MCU_CAN] -> Bus Creator1/3
  Bus Creator/1 -> Bus Creator1/4  "Controls"
  In5/1 -> Bus Creator1/5
  Bus Selector2/12 -> Data Type Conversion11/1  "<TrnsShftLvrPos>"
  Data Type Conversion11/1 -> Bus Creator/12  "ShftLvrPos"
  Bus Selector2/13 -> Data Type Conversion12/1  "<VehSpdAvgDrvn_kph>"
  Data Type Conversion12/1 -> Bus Creator/13  "VehSpdAvgDrvn_kph"
  Bus Selector2/14 -> Data Type Conversion13/1  "<AccPos_Perc>"
  Data Type Conversion13/1 -> Bus Creator/14  "AccPos_Perc"
  In6/1 -> Bus Creator1/6
  Memory/1 -> Data Type Conversion/1
  Memory1/1 -> Data Type Conversion1/1
  Memory2/1 -> Data Type Conversion10/1
  [ecm_CAN] -> Bus Creator1/7

== system P2_SIL_Model_Diag/Controller/HSC/Powertrain Manager/PowertrainSUSD ==
  note: //RWD.MaxShtdwnCurrent//
  note: //cal.Time.MCU.Restart.Time//
  note: //cal.Time.MCU.InvrtrRspns//
  HV_Bus_Status : Inport
  Sensors : Inport  Port=2
  Control : Inport  Port=3
  Bus Creator : BusCreator  Inputs=2
  Bus Creator1 : BusCreator  Inputs=4
  Bus Creator2 : BusCreator  Inputs=3
  Bus Selector : BusSelector  OutputSignals=from_CAN.fromHV_CAN.from_MCU.D6_Inverter_Enable_State,from_CAN.fromHV_CAN.from_MCU.D4_DC_Bus_Current
  Bus Selector1 : BusSelector  OutputSignals=ReadyToDrive,ReadyToCharge,HV Discharge
  Bus Selector2 : BusSelector  OutputSignals=EnableInverter
  Constant1 : Constant
  Constant2 : Constant  Value=0.5
  Constant3 : Constant
  Constant6 : Constant
  Crank Engine : Subsystem
  Data Type Conversion : DataTypeConversion  OutDataTypeStr=boolean
  Data Type Conversion1 : DataTypeConversion  OutDataTypeStr=boolean
  Data Type Conversion2 : DataTypeConversion  OutDataTypeStr=double
  From1 : From  Commented=on  GotoTag=Driver_Request  TagVisibility=global
  Motor Wake up / Shutdown : Stateflow chart  AncestorBlock=lib_PowertrainWUSD_Manager/PowertrainSUSD_Manager/Motor Wake up // Shutdown  TreatAsAtomicUnit=on
  Terminator : Terminator
  Terminator1 : Terminator
  Terminator2 : Terminator
  MCU_CAN : Outport
  MCU_Status : Outport  Port=2
  tag scope: ecm_CAN=global
  wires:
  Constant2/1 -> Motor Wake up / Shutdown/6(MaxShtdwnCrnt)
  Constant1/1 -> Motor Wake up / Shutdown/4(Inverter_Response_Time)
  Constant6/1 -> Motor Wake up / Shutdown/5(Restart_Time)
  Bus Selector/2 -> Motor Wake up / Shutdown/8(Motor_Current)  "<D4_DC_Bus_Current>"
  Motor Wake up / Shutdown/5(Inverter_Discharge) -> Data Type Conversion2/1
  Sensors/1 -> Crank Engine/1(Sensors), Bus Selector/1
  Bus Selector/1 -> Data Type Conversion1/1  "<D6_Inverter_Enable_State>"
  Data Type Conversion1/1 -> Motor Wake up / Shutdown/7(Inverter_Enabled)
  Bus Selector1/1 -> Motor Wake up / Shutdown/1(RdyToDrv)  "<ReadyToDrive>"
  Bus Selector1/2 -> Motor Wake up / Shutdown/2(RdyToChg)  "<ReadyToCharge>"
  Bus Selector1/3 -> Motor Wake up / Shutdown/3(HVDischarge)  "<HV Discharge>"
  Bus Creator/1 -> MCU_CAN/1  "MCU_CAN"
  HV_Bus_Status/1 -> Bus Selector1/1
  Data Type Conversion/1 -> Motor Wake up / Shutdown/9(CAN_Acc)
  Constant3/1 -> Data Type Conversion/1
  Motor Wake up / Shutdown/1(MCU_State) -> Bus Creator1/1  "MCU_State"
  Motor Wake up / Shutdown/2(MCU_ShtdwnRdy) -> Bus Creator1/2  "MCU_ShtdwnRdy"
  Motor Wake up / Shutdown/3(MCUFault) -> Bus Creator1/3  "MCUFault"
  Bus Creator1/1 -> MCU_Status/1  "MCU_Status"
  Control/1 -> Bus Selector2/1, Crank Engine/2(Control)
  Crank Engine/1(EngStatus) -> Bus Creator2/1, Terminator/1
  Crank Engine/2(EngCrankCmd) -> Bus Creator2/2, Terminator1/1
  Crank Engine/3(SysPwrMdOut) -> Bus Creator2/3, Terminator2/1
  Data Type Conversion2/1 -> Bus Creator/1  "Inverter_Discharge"
  Motor Wake up / Shutdown/6(Inverter_Enable) -> Bus Creator/2  "Inverter_Enable"
  Motor Wake up / Shutdown/4(MCU_Wake) -> Bus Creator1/4  "MCU Wake"
  Bus Selector2/1 -> Motor Wake up / Shutdown/10(EnableInverter)  "<EnableInverter>"
  Bus Creator2/1 -> [ecm_CAN]

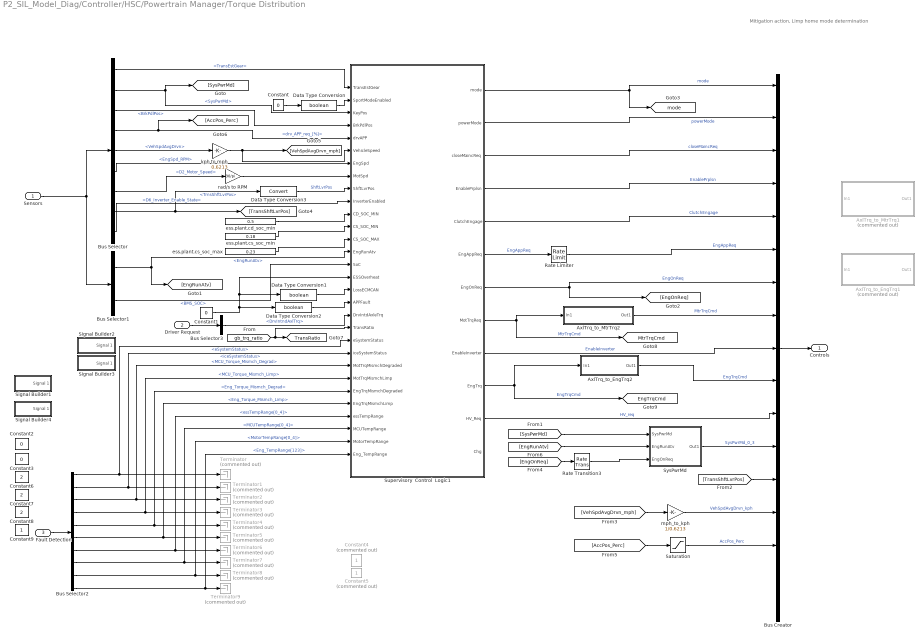
== system P2_SIL_Model_Diag/Controller/HSC/Powertrain Manager/Torque Distribution ==
  note: Mitigation action, Limp home mode determination
  Sensors : Inport
  Driver Request : Inport  Port=2
  Fault Detection : Inport  Port=3
  AxlTrq_to_EngTrq1 : Subsystem  Commented=on
  AxlTrq_to_EngTrq2 : Subsystem
  AxlTrq_to_MtrTrq1 : Subsystem  Commented=on
  AxlTrq_to_MtrTrq2 : Subsystem
  Bus Creator : BusCreator  Inputs=17
  Bus Selector : BusSelector  OutputSignals=from_CAN.fromVEH_CAN.from_TCM.TransEstGear,from_CAN.fromVEH_CAN.from_BCM.SysPwrMd,from_CAN.fromVEH_CAN.from_BCM.BrkPdlPos,from_Analog.drv_APP_req_[%],from_CAN.fromEBCAN.from_ECM.VehSpdAvgDrvn,from_CAN.fromEBCAN.from_ECM.EngSpd_RPM,from_CAN.fromHV_CAN.from_MCU.D2_Motor_Speed,from_CAN.fromVEH_CAN.from_TCM.TrnsShftLvrPos,from_CAN.fromHV_CAN.from_MCU.D6_Inverter_Enable_State
  Bus Selector1 : BusSelector  OutputSignals=from_CAN.fromEBCAN.from_ECM.EngRunAtv,from_CAN.fromHV_CAN.from_BMSHybrid.BMS_SOC
  Bus Selector2 : BusSelector  OutputSignals=eSystemDiagOut.eSystemStatus,iceSystemDiagOut.iceSystemStatus,CompSig.MCU_Torque_Mismch.MCU_Torque_Mismch_Degrad,CompSig.MCU_Torque_Mismch.MCU_Torque_Mismch_Limp,CompSig.EngTrqMismchType.Eng_Torque_Mismch_Degrad,CompSig.EngTrqMismchType.Eng_Torque_Mismch_Limp,CompSig.RawSig.ESS_SigDiag.essTempRange[0_4],CompSig.RawSig.Motor_SigDiag.MCUTempRange[0_4],CompSig.RawSig.Motor_SigDiag.MotorTempRange[0_4],CompSig.RawSig.Engine_SigDiag.Eng_TempRange[123]
  Bus Selector3 : BusSelector  OutputSignals=DrvIntndAxlTrq
  Constant{,1..3} (4 alike) : Constant  Value=0
  Constant4 : Constant  Commented=on
  Constant5 : Constant  Commented=on
  Constant6 : Constant  Value=2
  Constant7 : Constant  Value=2
  Constant8 : Constant  Value=2
  Constant9 : Constant
  Data Type Conversion : DataTypeConversion  OutDataTypeStr=boolean
  Data Type Conversion1 : DataTypeConversion  OutDataTypeStr=boolean
  Data Type Conversion2 : DataTypeConversion  OutDataTypeStr=boolean
  Data Type Conversion3 : DataTypeConversion
  Rate Limiter : RateLimiter  RisingSlewLimit=5/(1-tloop)  FallingSlewLimit=-5/(1-tloop)  SampleTimeMode=inherited
  Rate Transition3 : RateTransition
  Saturation : Saturate  UpperLimit=100  LowerLimit=0
  Signal Builder1 : Subsystem  Tag=STV Subsys  LoadFcn=sigbuilder_block('load');  StartFcn=sigbuilder_block('start');  StopFcn=sigbuilder_block('stop');  ClipboardFcn=sigbuilder_block('clipboard');  mask(Sigbuilder block){}
      mask help: Simulink:masks:SigbuilderBlock_MD
      mask init:
      | if ~strcmp(get_param(bdroot(gcbh),'SimulationStatus'),'stopped') tuvar = sigbuilder_block('maskInit'); end
      settings: CopyFcn=sigbuilder_block('copy');  DeleteFcn=sigbuilder_block('delete');  ModelCloseFcn=sigbuilder_block('modelClose');  PreSaveFcn=sigbuilder_block('preSave');  PauseFcn=sigbuilder_block('pause');  ContinueFcn=sigbuilder_block('continue');  NameChangeFcn=sigbuilder_block('namechange');  OpenFcn=sigbuilder_block('open',[202.8 56.4 550.8 400.2 ]);  CloseFcn=sigbuilder_block('close');
      mask Display: plot(0, 0, 100, 100,[2, 2, 32, 32, 2], [68, 8, 8, 68, 68],[32, 2], [38, 38], [32, 19, 2],[53, 60, 44], [32, 17, 17, 2],[16, 16, 31, 31]);txt = getActiveGroup(gcbh);text(2, 100, txt,'verticalAlignment', 'top');
  Signal Builder2 : Subsystem  Tag=STV Subsys  LoadFcn=sigbuilder_block('load');  StartFcn=sigbuilder_block('start');  StopFcn=sigbuilder_block('stop');  ClipboardFcn=sigbuilder_block('clipboard');  mask(Sigbuilder block){}
      mask help: Simulink:masks:SigbuilderBlock_MD
      mask init:
      | if ~strcmp(get_param(bdroot(gcbh),'SimulationStatus'),'stopped') tuvar = sigbuilder_block('maskInit'); end
      settings: CopyFcn=sigbuilder_block('copy');  DeleteFcn=sigbuilder_block('delete');  ModelCloseFcn=sigbuilder_block('modelClose');  PreSaveFcn=sigbuilder_block('preSave');  PauseFcn=sigbuilder_block('pause');  ContinueFcn=sigbuilder_block('continue');  NameChangeFcn=sigbuilder_block('namechange');  OpenFcn=sigbuilder_block('open',[184.8 48 550.8 400.2 ]);  CloseFcn=sigbuilder_block('close');
      mask Display: plot(0, 0, 100, 100,[2, 2, 32, 32, 2], [68, 8, 8, 68, 68],[32, 2], [38, 38], [32, 19, 2],[53, 60, 44], [32, 17, 17, 2],[16, 16, 31, 31]);txt = getActiveGroup(gcbh);text(2, 100, txt,'verticalAlignment', 'top');
  Signal Builder3 : Subsystem  Tag=STV Subsys  LoadFcn=sigbuilder_block('load');  StartFcn=sigbuilder_block('start');  StopFcn=sigbuilder_block('stop');  ClipboardFcn=sigbuilder_block('clipboard');  mask(Sigbuilder block){}
      mask help: Simulink:masks:SigbuilderBlock_MD
      mask init:
      | if ~strcmp(get_param(bdroot(gcbh),'SimulationStatus'),'stopped') tuvar = sigbuilder_block('maskInit'); end
      settings: CopyFcn=sigbuilder_block('copy');  DeleteFcn=sigbuilder_block('delete');  ModelCloseFcn=sigbuilder_block('modelClose');  PreSaveFcn=sigbuilder_block('preSave');  PauseFcn=sigbuilder_block('pause');  ContinueFcn=sigbuilder_block('continue');  NameChangeFcn=sigbuilder_block('namechange');  OpenFcn=sigbuilder_block('open',[416.4 91.8 550.8 400.2 ]);  CloseFcn=sigbuilder_block('close');
      mask Display: plot(0, 0, 100, 100,[2, 2, 32, 32, 2], [68, 8, 8, 68, 68],[32, 2], [38, 38], [32, 19, 2],[53, 60, 44], [32, 17, 17, 2],[16, 16, 31, 31]);txt = getActiveGroup(gcbh);text(2, 100, txt,'verticalAlignment', 'top');
  Signal Builder4 : Subsystem  Tag=STV Subsys  LoadFcn=sigbuilder_block('load');  StartFcn=sigbuilder_block('start');  StopFcn=sigbuilder_block('stop');  ClipboardFcn=sigbuilder_block('clipboard');  mask(Sigbuilder block){}
      mask help: Simulink:masks:SigbuilderBlock_MD
      mask init:
      | if ~strcmp(get_param(bdroot(gcbh),'SimulationStatus'),'stopped') tuvar = sigbuilder_block('maskInit'); end
      settings: CopyFcn=sigbuilder_block('copy');  DeleteFcn=sigbuilder_block('delete');  ModelCloseFcn=sigbuilder_block('modelClose');  PreSaveFcn=sigbuilder_block('preSave');  PauseFcn=sigbuilder_block('pause');  ContinueFcn=sigbuilder_block('continue');  NameChangeFcn=sigbuilder_block('namechange');  OpenFcn=sigbuilder_block('open',[416.4 91.8 550.8 400.2 ]);  CloseFcn=sigbuilder_block('close');
      mask Display: plot(0, 0, 100, 100,[2, 2, 32, 32, 2], [68, 8, 8, 68, 68],[32, 2], [38, 38], [32, 19, 2],[53, 60, 44], [32, 17, 17, 2],[16, 16, 31, 31]);txt = getActiveGroup(gcbh);text(2, 100, txt,'verticalAlignment', 'top');
  Supervisory  Control  Logic1 : Stateflow chart  TreatAsAtomicUnit=on
  SysPwrMd : Subsystem
  Terminator{,1..9} (10 alike) : Terminator  Commented=on
  ess.plant.cd_soc_min : Constant  Value=0.5
  ess.plant.cs_soc_max : Constant  Value=0.23
  ess.plant.cs_soc_min : Constant  Value=0.18
  kph to mph : Gain  Gain=0.6213
  mph_to_kph : Gain  Gain=1/0.6213
  rad/s to RPM : Gain  Gain=30/pi
  Controls : Outport
  tag scope: EngTrqCmd=global, MtrTrqCmd=global, TransRatio=global, mode=global
  wires:
  Sensors/1 -> Bus Selector1/1, Bus Selector/1
  Bus Selector/1 -> Supervisory  Control  Logic1/1(TransEstGear)  "<TransEstGear>"
  Bus Selector/2 -> Supervisory  Control  Logic1/3(KeyPos), [SysPwrMd]  "<SysPwrMd>"
  Bus Selector/3 -> Supervisory  Control  Logic1/4(BrkPdlPos)  "<BrkPdlPos>"
  Bus Selector/4 -> [AccPos_Perc], Supervisory  Control  Logic1/5(drvAPP)  "<drv_APP_req_[%]>"
  Bus Selector/5 -> kph to mph/1  "<VehSpdAvgDrvn>"
  Bus Selector/6 -> Supervisory  Control  Logic1/7(EngSpd)  "<EngSpd_RPM>"
  Bus Selector/7 -> rad/s to RPM/1  "<D2_Motor_Speed>"
  Bus Selector/9 -> Supervisory  Control  Logic1/10(InverterEnabled)  "<D6_Inverter_Enable_State>"
  Bus Selector1/1 -> [EngRunAtv], Supervisory  Control  Logic1/14(EngRunAtv)  "<EngRunAtv>"
  Bus Selector1/2 -> Supervisory  Control  Logic1/15(SoC)  "<BMS_SOC>"
  Constant1/1 -> Data Type Conversion1/1, Supervisory  Control  Logic1/16(ESSOverheat), Data Type Conversion2/1
  ess.plant.cd_soc_min/1 -> Supervisory  Control  Logic1/11(CD_SOC_MIN)
  ess.plant.cs_soc_min/1 -> Supervisory  Control  Logic1/12(CS_SOC_MIN)
  ess.plant.cs_soc_max/1 -> Supervisory  Control  Logic1/13(CS_SOC_MAX)
  Supervisory  Control  Logic1/7(EngOnReq) -> [EngOnReq], Bus Creator/7  "EngOnReq"
  Supervisory  Control  Logic1/9(EnableInverter) -> Bus Creator/9  "EnableInverter"
  Supervisory  Control  Logic1/6(EngAppReq) -> Rate Limiter/1  "EngAppReq"
  Supervisory  Control  Logic1/4(EnablePrplsn) -> Bus Creator/4  "EnablePrplsn"
  Supervisory  Control  Logic1/3(closeMaincReq) -> Bus Creator/3  "closeMaincReq"
  Supervisory  Control  Logic1/2(powerMode) -> Bus Creator/2  "powerMode"
  Supervisory  Control  Logic1/1(mode) -> [mode], Bus Creator/1  "mode"
  [EngOnReq] -> Rate Transition3/1
  [EngRunAtv] -> SysPwrMd/2(EngRunAtv)
  [SysPwrMd] -> SysPwrMd/1(SysPwrMd)
  Constant/1 -> Data Type Conversion/1
  Data Type Conversion/1 -> Supervisory  Control  Logic1/2(SportModeEnabled)
  Data Type Conversion1/1 -> Supervisory  Control  Logic1/17(LossECMCAN)
  Data Type Conversion2/1 -> Supervisory  Control  Logic1/18(APPFault)
  Data Type Conversion3/1 -> Supervisory  Control  Logic1/9(ShftLvrPos)  "ShftLvrPos"
  Bus Selector/8 -> Data Type Conversion3/1, [TransShftLvrPos]  "<TrnsShftLvrPos>"
  kph to mph/1 -> Supervisory  Control  Logic1/6(VehicleSpeed), [VehSpdAvgDrvn_mph]
  rad/s to RPM/1 -> Supervisory  Control  Logic1/8(MotSpd)
  Bus Creator/1 -> Controls/1
  Supervisory  Control  Logic1/10(EngTrq) -> AxlTrq_to_EngTrq2/1(In1), [EngTrqCmd]  "EngTrqCmd"
  [gb_trq_ratio] -> Supervisory  Control  Logic1/20(TransRatio), [TransRatio]
  SysPwrMd/1(Out1) -> Bus Creator/12  "SysPwrMd_0_3"
  Supervisory  Control  Logic1/11(HV_Req) -> Bus Creator/11  "HV_req"
  [TransShftLvrPos] -> Bus Creator/13
  [VehSpdAvgDrvn_mph] -> mph_to_kph/1
  mph_to_kph/1 -> Bus Creator/14  "VehSpdAvgDrvn_kph"
  [AccPos_Perc] -> Saturation/1
  Saturation/1 -> Bus Creator/15  "AccPos_Perc"
  Driver Request/1 -> Bus Selector3/1
  Bus Selector3/1 -> Supervisory  Control  Logic1/19(DrvIntdAxleTrq)  "<DrvIntndAxlTrq>"
  Rate Transition3/1 -> SysPwrMd/3(EngOnReq)
  Supervisory  Control  Logic1/5(ClutchEngage) -> Bus Creator/5  "ClutchEngage"
  Rate Limiter/1 -> Bus Creator/6  "EngAppReq"
  Supervisory  Control  Logic1/8(MotTrqReq) -> [MtrTrqCmd], AxlTrq_to_MtrTrq2/1(In1)  "MtrTrqCmd"
  AxlTrq_to_MtrTrq2/1(Out1) -> Bus Creator/8  "MtrTrqCmd"
  AxlTrq_to_EngTrq2/1(Out1) -> Bus Creator/10  "EngTrqCmd"
  Fault Detection/1 -> Bus Selector2/1
  Bus Selector2/1 -> Terminator/1, Supervisory  Control  Logic1/21(eSystemStatus)  "<eSystemStatus>"
  Bus Selector2/3 -> Terminator2/1, Supervisory  Control  Logic1/23(MotTrqMismchDegraded)  "<MCU_Torque_Mismch_Degrad>"
  Bus Selector2/4 -> Terminator3/1, Supervisory  Control  Logic1/24(MotTrqMismchLimp)  "<MCU_Torque_Mismch_Limp>"
  Bus Selector2/5 -> Terminator4/1, Supervisory  Control  Logic1/25(EngTrqMismchDegraded)  "<Eng_Torque_Mismch_Degrad>"
  Bus Selector2/6 -> Terminator5/1, Supervisory  Control  Logic1/26(EngTrqMismchLimp)  "<Eng_Torque_Mismch_Limp>"
  Bus Selector2/7 -> Supervisory  Control  Logic1/27(essTempRange), Terminator6/1  "<essTempRange[0_4]>"
  Bus Selector2/8 -> Terminator7/1, Supervisory  Control  Logic1/28(MCUTempRange)  "<MCUTempRange[0_4]>"
  Bus Selector2/9 -> Terminator8/1, Supervisory  Control  Logic1/29(MotorTempRange)  "<MotorTempRange[0_4]>"
  Bus Selector2/2 -> Terminator1/1, Supervisory  Control  Logic1/22(iceSystemStatus)  "<iceSystemStatus>"
  Bus Selector2/10 -> Terminator9/1, Supervisory  Control  Logic1/30(Eng_TempRange)  "<Eng_TempRange[123]>"

== system P2_SIL_Model_Diag/Plant Actuators/CAN/EBCAN/BMS_Antrieb ==
  In1 : Inport
  Bus Selector : BusSelector  OutputSignals=BMS_CAN.BMS_Hybrid
  Out1 : Outport
  wires:
  Bus Selector/1 -> Out1/1  "<BMS_Hybrid>"
  In1/1 -> Bus Selector/1

== system P2_SIL_Model_Diag/Plant Actuators/CAN/EBCAN/ECM ==
  In1 : Inport
  Bus Selector : BusSelector  OutputSignals=ECM_CAN
  Out1 : Outport
  wires:
  Bus Selector/1 -> Out1/1  "<ECM_CAN>"
  In1/1 -> Bus Selector/1

== system P2_SIL_Model_Diag/Plant Actuators/CAN/HV_CAN/APM ==
  In1 : Inport
  Bus Selector : BusSelector  OutputSignals=APM_CAN
  Out1 : Outport
  wires:
  Bus Selector/1 -> Out1/1  "<APM_CAN>"
  In1/1 -> Bus Selector/1
